simulink model "Maglev_PID_model"  (R2021a)
settings: Solver=VariableStepAuto  StartTime=0.0  StopTime=10.0  RelTol=1e-3
libraries: pid_lib x1
settings Model: Creator=user  LastModifiedBy=user

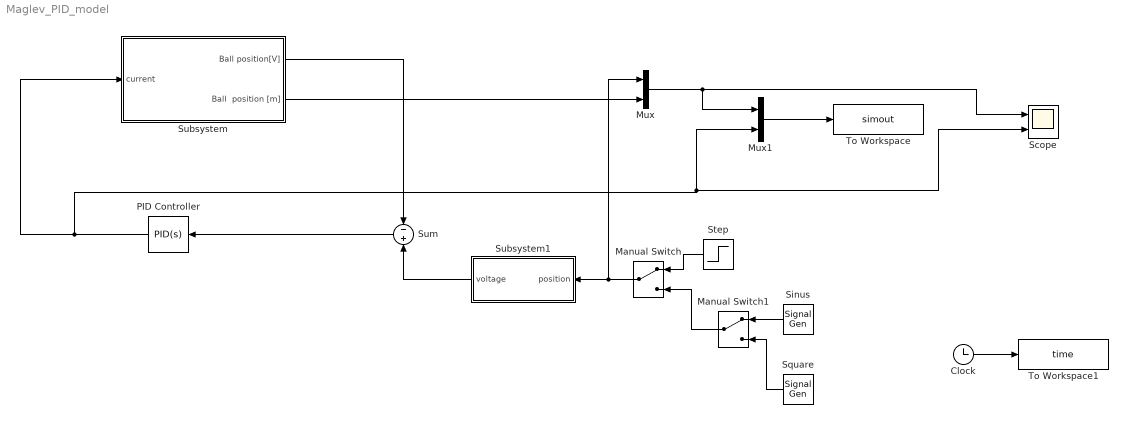
== system Maglev_PID_model ==
  Clock : Clock
  Manual Switch : ManualSwitch
  Manual Switch1 : ManualSwitch
  Mux : Mux  Inputs=2
  Mux1 : Mux  Inputs=2
  PID Controller : pid_lib/PID Controller  Controller=PID  Form=Parallel  TimeDomain=Continuous-time  UseExternalTs=off  SampleTime=-1  IntegratorMethod=Forward Euler  FilterMethod=Forward Euler  ControllerParametersSource=internal  P=3  I=0.75  D=0.3  UseFilter=on  N=100  TunerSelectOption=Transfer Function Based (PID Tuner App)  InitialConditionSource=internal  InitialConditionForIntegrator=0  InitialConditionForFilter=0  DifferentiatorICPrevScaledInput=0  ExternalReset=none  TrackingMode=off  Kt=1  LimitOutput=off  SatLimitsSource=internal  UpperSaturationLimit=inf  LowerSaturationLimit=-inf  LinearizeAsGain=on  AntiWindupMode=none  Kb=1  POutMin=[]  POutMax=[]  IOutMin=[]  IOutMax=[]  DOutMin=[]  DOutMax=[]  NOutMin=[]  NOutMax=[]  SumOutMin=[]  SumOutMax=[]  SaturationOutMin=[]  SaturationOutMax=[]  PParamMin=[]  PParamMax=[]  IParamMin=[]  IParamMax=[]  DParamMin=[]  DParamMax=[]  NParamMin=[]  NParamMax=[]  KbParamMin=[]  KbParamMax=[]  KtParamMin=[]  KtParamMax=[]  KbOutMin=[]  KbOutMax=[]  KtOutMin=[]  KtOutMax=[]  IntegratorOutMin=[]  IntegratorOutMax=[]  FilterOutMin=[]  FilterOutMax=[]  SumI1OutMin=[]  SumI1OutMax=[]  SumI2OutMin=[]  SumI2OutMax=[]  SumI3OutMin=[]  SumI3OutMax=[]  SumI4OutMin=[]  SumI4OutMax=[]  SumDOutMin=[]  SumDOutMax=[]  DifferentiatorOutMin=[]  DifferentiatorOutMax=[]  FilterDiffOutCoefMin=[]  FilterDiffOutCoefMax=[]  ReciprocalOutMin=[]  ReciprocalOutMax=[]  SumDenOutMin=[]  SumDenOutMax=[]  SumNumOutMin=[]  SumNumOutMax=[]  DivideOutMin=[]  DivideOutMax=[]  UdiffTsProdOutMin=[]  UdiffTsProdOutMax=[]  NTsProdOutMin=[]  NTsProdOutMax=[]  UintegralTsProdOutMin=[]  UintegralTsProdOutMax=[]  UngainTsProdOutMin=[]  UngainTsProdOutMax=[]  IntegratorContinuousStateAttributes=''  IntegratorStateMustResolveToSignalObject=off  IntegratorRTWStateStorageClass=Auto  FilterContinuousStateAttributes=''  FilterStateMustResolveToSignalObject=off  FilterRTWStateStorageClass=Auto  ParallelPVariant=InternalParameters  IdealPVariant=Disabled  IVariant=InternalParameters  DVariant=InternalParameters  IntegratorVariant=Continuous  SatVariant=Disabled  AWVariant=Passthrough  PCopyVariant=Disabled  TRVariant=Disabled  FdbkBlocksVariant=Forward  IdealPFdbkVariant=Disabled  SatFdbkVariant=Disabled  DerivativeFilterVariant=ContFilter  NVariant=InternalParameters  NCopyVariant=Disabled  FilterICVariant=InternalICsFilter  IntegratorICVariant=InternalICs  ExternalResetVariant=Disabled  TRSumVariant=Passthrough  SumFdbkVariant=Disabled  SumVariant=Sum_PID  TsampFilterVariant=InternalTs  TsampNgainVariant=Passthrough  TsampIntegralVariant=Passthrough  ExternalSaturationOutDataTypeStr=Inherit: Same as second input
  Scope : Scope  NumInputPorts=2
  Sinus : SignalGenerator  Units=rad/sec
  Square : SignalGenerator  Units=rad/sec
  Step : Step  SampleTime=0
  Subsystem : Subsystem
  Subsystem1 : Subsystem
  Sum : Sum  Inputs=-+
  To Workspace : ToWorkspace  VariableName=simout  SampleTime=-1
      settings: Save2DSignal=2-D array (concatenate along first dimension)
  To Workspace1 : ToWorkspace  VariableName=time  SampleTime=-1
      settings: Save2DSignal=2-D array (concatenate along first dimension)
  wires:
  Subsystem/1(Ball position[V]) -> Sum/1
  Subsystem/2(Ball  position [m]) -> Mux/2
  Subsystem1/1(voltage) -> Sum/2
  Sum/1 -> PID Controller/1
  Mux1/1 -> To Workspace/1
  Clock/1 -> To Workspace1/1
  Manual Switch/1 -> Mux/1, Subsystem1/1(position)
  Manual Switch1/1 -> Manual Switch/2
  Mux/1 -> Mux1/1, Scope/1
  Sinus/1 -> Manual Switch1/1
  Square/1 -> Manual Switch1/2
  Step/1 -> Manual Switch/1
  PID Controller/1 -> Mux1/2, Scope/2, Subsystem/1(current)

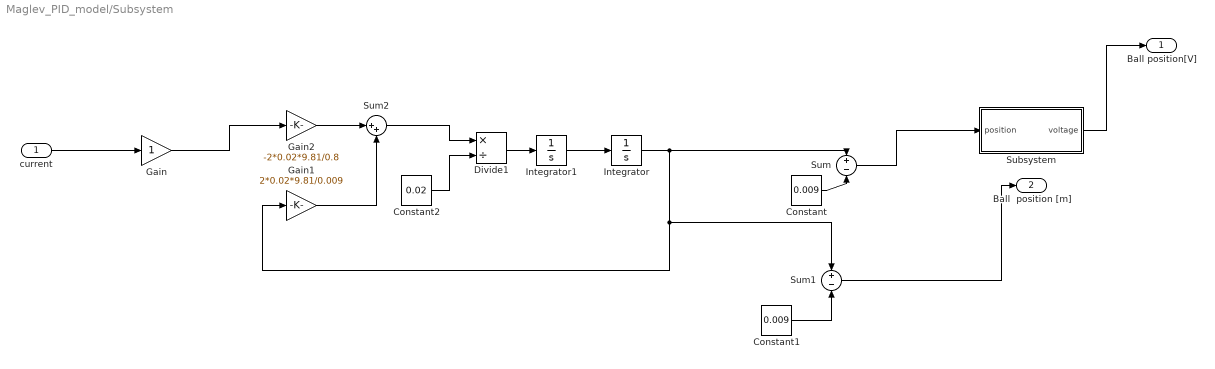
== system Maglev_PID_model/Subsystem ==
  current : Inport
  Constant : Constant  Value=0.009
  Constant1 : Constant  Value=0.009
  Constant2 : Constant  Value=0.02
  Divide1 : Product  Inputs=*/
  Gain : Gain
  Gain1 : Gain  Gain=2*0.02*9.81/0.009
  Gain2 : Gain  Gain=-2*0.02*9.81/0.8
  Integrator : Integrator
  Integrator1 : Integrator
  Subsystem : Subsystem
  Sum : Sum  Inputs=+-
  Sum1 : Sum  Inputs=+-
  Sum2 : Sum  Inputs=|++
  Ball position[V] : Outport
  Ball  position [m] : Outport  Port=2
  wires:
  current/1 -> Gain/1
  Gain/1 -> Gain2/1
  Integrator1/1 -> Integrator/1
  Integrator/1 -> Gain1/1, Sum1/1, Sum/1
  Constant/1 -> Sum/2
  Constant1/1 -> Sum1/2
  Sum/1 -> Subsystem/1(position)
  Sum1/1 -> Ball  position [m]/1
  Subsystem/1(voltage) -> Ball position[V]/1
  Divide1/1 -> Integrator1/1
  Constant2/1 -> Divide1/2
  Gain2/1 -> Sum2/1
  Gain1/1 -> Sum2/2
  Sum2/1 -> Divide1/1

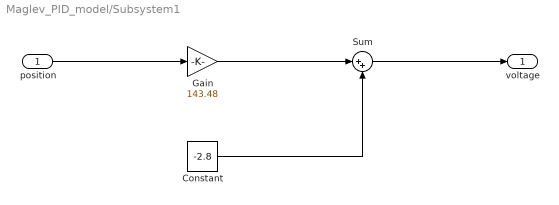
== system Maglev_PID_model/Subsystem1 ==
  position : Inport  Unit=m
  Constant : Constant  Value=-2.8
  Gain : Gain  Gain=143.48
  Sum : Sum  Inputs=|++
  voltage : Outport  Unit=V
  wires:
  Gain/1 -> Sum/1
  Constant/1 -> Sum/2
  Sum/1 -> voltage/1
  position/1 -> Gain/1

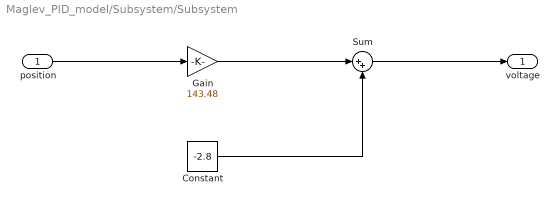
== system Maglev_PID_model/Subsystem/Subsystem ==
  position : Inport  Unit=m
  Constant : Constant  Value=-2.8
  Gain : Gain  Gain=143.48
  Sum : Sum  Inputs=|++
  voltage : Outport  Unit=V
  wires:
  Gain/1 -> Sum/1
  Constant/1 -> Sum/2
  Sum/1 -> voltage/1
  position/1 -> Gain/1
